simulink model "model_2"  (R2023b)
settings: Solver=VariableStepAuto  StartTime=0.0  StopTime=Tmdl  RelTol=1e-3
undefined symbols (not defined in the file): Ad, Bd, Bdf, C, Gf, Gg, Hf, Hg, Koc, L, Lf, Lg, Mg, T, x_hat_initial, x_initial, xi_initial, xif_initial
settings Model: Creator=deniskirbaba  LastModifiedBy=deniskirbaba

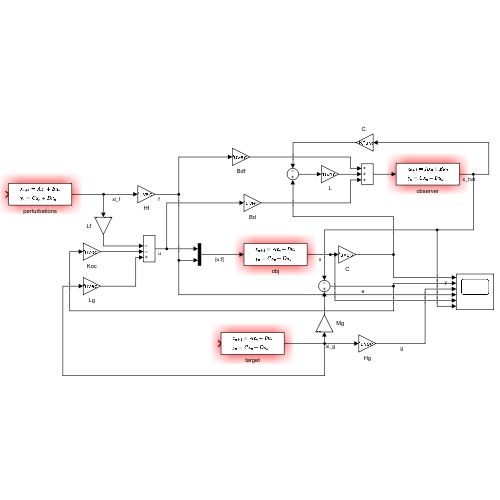
[thumbnail: Simulink's stored preview of the top-level diagram]
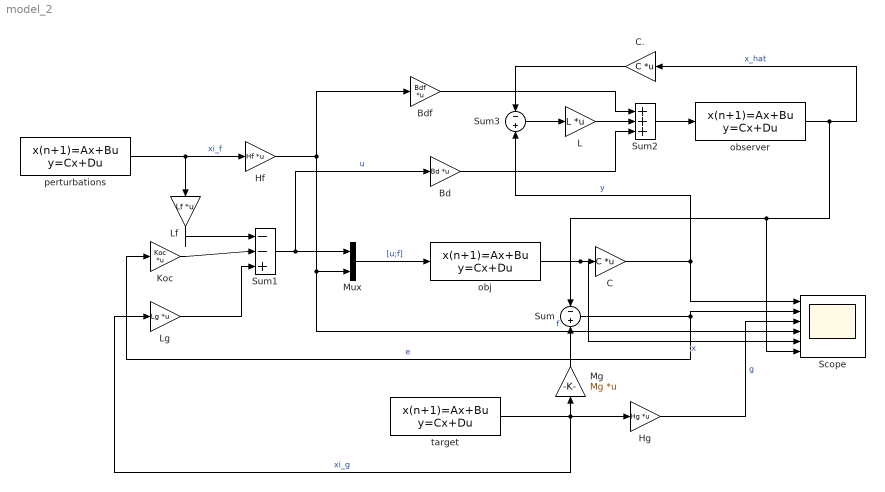
== system model_2 ==
  Bd : Gain  Gain=Bd  Multiplication=Matrix(K*u) (u vector)
  Bdf : Gain  Gain=Bdf  Multiplication=Matrix(K*u) (u vector)
  C : Gain  Gain=C  Multiplication=Matrix(K*u) (u vector)
  C. : Gain  Gain=C  Multiplication=Matrix(K*u) (u vector)
  Hf : Gain  Gain=Hf  Multiplication=Matrix(K*u) (u vector)
  Hg : Gain  Gain=Hg  Multiplication=Matrix(K*u) (u vector)
  Koc : Gain  Gain=Koc  Multiplication=Matrix(K*u) (u vector)
  L : Gain  Gain=L  Multiplication=Matrix(K*u) (u vector)
  Lf : Gain  Gain=Lf  Multiplication=Matrix(K*u) (u vector)
  Lg : Gain  Gain=Lg  Multiplication=Matrix(K*u) (u vector)
  Mg : Gain  Gain=Mg  Multiplication=Matrix(K*u) (u vector)
  Mux : Mux  Inputs=2
  Scope : Scope  NumInputPorts=6
  Sum : Sum  Inputs=-+
  Sum1 : Sum  Inputs=|--+
  Sum2 : Sum  Inputs=+++
  Sum3 : Sum  Inputs=-|+
  obj : DiscreteStateSpace  A=Ad  B=[Bd Bdf]  C=eye(2)  D=[0 0;0 0]  InitialCondition=x_initial  SampleTime=T
  observer : DiscreteStateSpace  A=Ad  B=eye(2)  C=eye(2)  D=[0 0;0 0]  InitialCondition=x_hat_initial  SampleTime=T
  perturbations : DiscreteStateSpace  A=Gf  B=[0;0]  C=eye(2)  D=[0;0]  InitialCondition=xif_initial  SampleTime=T
  target : DiscreteStateSpace  A=Gg  B=zeros([2 1])  C=eye(2)  D=[0;0]  InitialCondition=xi_initial  SampleTime=T
  wires:
  target/1 -> Hg/1, Mg/1, Lg/1  "xi_g"
  obj/1 -> Scope/5, C/1  "x"
  C/1 -> Scope/1, Sum3/2  "y"
  Sum/1 -> Scope/2, Koc/1  "e"
  Hg/1 -> Scope/3  "g"
  Koc/1 -> Sum1/2
  Lg/1 -> Sum1/3
  Sum1/1 -> Bd/1, Mux/1  "u"
  Mg/1 -> Sum/2
  perturbations/1 -> Lf/1, Hf/1  "xi_f"
  Hf/1 -> Bdf/1, Scope/4, Mux/2  "f"
  Lf/1 -> Sum1/1
  Mux/1 -> obj/1  "[u;f]"
  Sum2/1 -> observer/1
  Bd/1 -> Sum2/3
  observer/1 -> C./1, Scope/6, Sum/1  "x_hat"
  L/1 -> Sum2/2
  Sum3/1 -> L/1
  C./1 -> Sum3/1
  Bdf/1 -> Sum2/1
